simulink model "DisplayModel_Step3_start_harness"  (R2013b)
settings: Solver=FixedStepDiscrete  StartTime=0.0  StopTime=10.0  FixedStep=0.2  RelTol=1e-3
undefined symbols (not defined in the file): sigbuilder_block
libraries: simulink x1
settings Model: SldvGeneratedHarnessModel=TestUnitModel=DisplayModel_Step3_start|  CovMetricSettings=dcmoe  CovHTMLOptions=-aTS=1 -bRG=1 -bTC=0 -hTR=0 -nFC=0 -scm=1 -bcm=1  CovModelRefEnable=on  CovExternalEMLEnable=on  Creator=siddhars  LastModifiedBy=hualongy
settings DataIOCC: SaveFormat=StructureWithTime
settings OptimizationCC: ExpressionDepthLimit=2147483647  OptimizeModelRefInitCode=on  LifeSpan=1
settings DebuggingCC: InheritedTsInSrcMsg=none  StateNameClashWarn=warning
settings RTWCC: SystemTargetFile=ert.tlc  TemplateMakefile=ert_default_tmf  Description=Embedded Coder  ProcessScript=ert_make_rtw_hook  PortableWordSizes=on
settings CodeAppCC: IgnoreCustomStorageClasses=off  CustomSymbolStrType=$N$R$M  InternalIdentifier=Classic
settings ERTTargetCC: CodeReplacementLibrary=ANSI_C  GenerateSampleERTMain=on  ERTCustomFileTemplate=example_file_process.tlc
settings ConfigComp: Description=Design Verifier Custom Configuration Component  DVModelCoverageObjectives=MCDC  DVMaxTestCaseSteps=500  DVTestSuiteOptimization=CombinedObjectives (Nonlinear Extended)  DVSaveHarnessModel=on  DVModelReferenceHarness=on

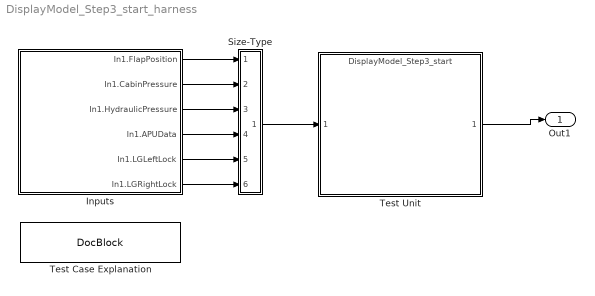
== system DisplayModel_Step3_start_harness ==
  Inputs : Subsystem  Tag=STV Subsys  LoadFcn=sigbuilder_block('load',[49.5 50.25 519.75 399.75 ]);  StartFcn=sigbuilder_block('start');  StopFcn=sigbuilder_block('stop');  ClipboardFcn=sigbuilder_block('clipboard');  mask(Sigbuilder block){}
      mask init:
      | if ~strcmp(get_param(bdroot(gcb),'SimulationStatus'),'stopped'),tuvar = sigbuilder_block('maskInit'); end
      settings: CopyFcn=sigbuilder_block('copy');  DeleteFcn=sigbuilder_block('delete');  ModelCloseFcn=sigbuilder_block('modelClose');  PreSaveFcn=sigbuilder_block('preSave');  PauseFcn=sigbuilder_block('pause');  ContinueFcn=sigbuilder_block('continue');  NameChangeFcn=sigbuilder_block('namechange');  OpenFcn=sigbuilder_block('open');  CloseFcn=sigbuilder_block('close');
      mask Display: plot(0, 0, 100, 100,[2, 2, 32, 32, 2], [68, 8, 8, 68, 68],[32, 2], [38, 38], [32, 19, 2],[53, 60, 44], [32, 17, 17, 2],[16, 16, 31, 31]);txt = getActiveGroup(gcbh);text(2, 100, txt,'verticalAlignment', 'top');
  Size-Type : Subsystem
  Test Case Explanation : simulink/Model-Wide Utilities/DocBlock  DocumentType=Text
  Test Unit : ModelReference  ModelNameDialog=DisplayModel_Step3_start  SimulationMode=Normal  ModelReferenceVersion=1.64  CopyOfModelName=DisplayModel_Step3_start  DefaultDataLogging=on
  Out1 : Outport
  wires:
  Inputs/1(In1.FlapPosition) -> Size-Type/1(In1)
  Inputs/2(In1.CabinPressure) -> Size-Type/2(In2)
  Inputs/3(In1.HydraulicPressure) -> Size-Type/3(In3)
  Inputs/4(In1.APUData) -> Size-Type/4(In4)
  Inputs/5(In1.LGLeftLock) -> Size-Type/5(In5)
  Inputs/6(In1.LGRightLock) -> Size-Type/6(In6)
  Size-Type/1(Out1) -> Test Unit/1
  Test Unit/1 -> Out1/1

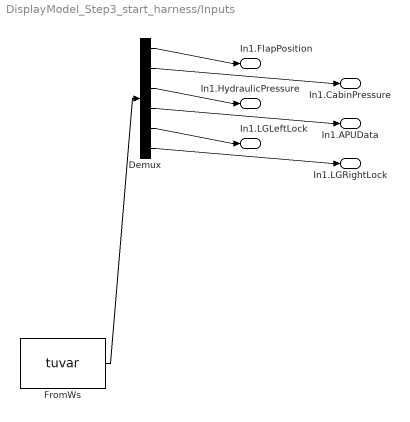
== system DisplayModel_Step3_start_harness/Inputs ==
  Demux : Demux  Tag=STV Demux  Outputs=6
  FromWs : FromWorkspace  Tag=STV FromWs  VariableName=tuvar  SampleTime=0
      SigBuilderData=|
      | dataSet.timeRange = [0 0.2]
      | dataSet.name = 'Test Case 1'
      | sbobj.Name = 'Signal Builder'
      | sbobj.Groups.Name = 'Test Case 1'
      | sbobj.Groups.Signals(1).Name = 'In1.FlapPosition'
      | sbobj.Groups.Signals(1).XData = [0 0.2]
      | sbobj.Groups.Signals(1).YData = [0 0]
      | sbobj.Groups.Signals(2).Name = 'In1.CabinPressure'
      | sbobj.Groups.Signals(2).XData = [0 0.2]
      | sbobj.Groups.Signals(2).YData = [0 0]
      | sbobj.Groups.Signals(3).Name = 'In1.HydraulicPressure'
      | sbobj.Groups.Signals(3).XData = [0 0.2]
      | sbobj.Groups.Signals(3).YData = [0 0]
      | sbobj.Groups.Signals(4).Name = 'In1.APUData'
      | sbobj.Groups.Signals(4).XData = [0 0.2]
      | sbobj.Groups.Signals(4).YData = [0 0]
      | sbobj.Groups.Signals(5).Name = 'In1.LGLeftLock'
      | sbobj.Groups.Signals(5).XData = [0 0.2]
      | sbobj.Groups.Signals(5).YData = [0 0]
      | sbobj.Groups.Signals(6).Name = 'In1.LGRightLock'
      | sbobj.Groups.Signals(6).XData = [0 0.2]
      | sbobj.Groups.Signals(6).YData = [0 0]
      | sbobj.Groups.TimeRange = [0 0.2]
  In1.FlapPosition : Outport  Tag=STV Outport
  In1.CabinPressure : Outport  Tag=STV Outport  Port=2
  In1.HydraulicPressure : Outport  Tag=STV Outport  Port=3
  In1.APUData : Outport  Tag=STV Outport  Port=4
  In1.LGLeftLock : Outport  Tag=STV Outport  Port=5
  In1.LGRightLock : Outport  Tag=STV Outport  Port=6
  wires:
  FromWs/1 -> Demux/1
  Demux/1 -> In1.FlapPosition/1
  Demux/2 -> In1.CabinPressure/1
  Demux/3 -> In1.HydraulicPressure/1
  Demux/4 -> In1.APUData/1
  Demux/5 -> In1.LGLeftLock/1
  Demux/6 -> In1.LGRightLock/1

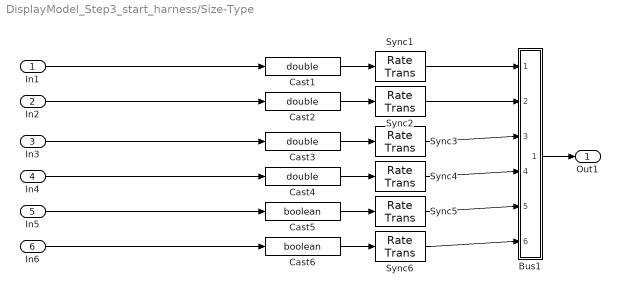
== system DisplayModel_Step3_start_harness/Size-Type ==
  In1 : Inport
  In2 : Inport  Port=2
  In3 : Inport  Port=3
  In4 : Inport  Port=4
  In5 : Inport  Port=5
  In6 : Inport  Port=6
  Bus1 : Subsystem
  Cast{1..4} (4 alike) : DataTypeConversion  OutDataTypeStr=double  SaturateOnIntegerOverflow=on  RndMeth=Zero
  Cast5 : DataTypeConversion  OutDataTypeStr=boolean  SaturateOnIntegerOverflow=on  RndMeth=Zero
  Cast6 : DataTypeConversion  OutDataTypeStr=boolean  SaturateOnIntegerOverflow=on  RndMeth=Zero
  Sync{1..6} (6 alike) : RateTransition  OutPortSampleTime=[0.20000000000000001,0]
  Out1 : Outport
  wires:
  In1/1 -> Cast1/1
  Cast1/1 -> Sync1/1
  In2/1 -> Cast2/1
  Cast2/1 -> Sync2/1
  In3/1 -> Cast3/1
  Cast3/1 -> Sync3/1
  In4/1 -> Cast4/1
  Cast4/1 -> Sync4/1
  In5/1 -> Cast5/1
  Cast5/1 -> Sync5/1
  In6/1 -> Cast6/1
  Cast6/1 -> Sync6/1
  Sync1/1 -> Bus1/1(In1(1).FlapPosition)
  Sync2/1 -> Bus1/2(In1(1).CabinPressure)
  Sync3/1 -> Bus1/3(In1(1).HydraulicPressure)
  Sync4/1 -> Bus1/4(In1(1).APUData)
  Sync5/1 -> Bus1/5(In1(1).LGLeftLock)
  Sync6/1 -> Bus1/6(In1(1).LGRightLock)
  Bus1/1(Out) -> Out1/1

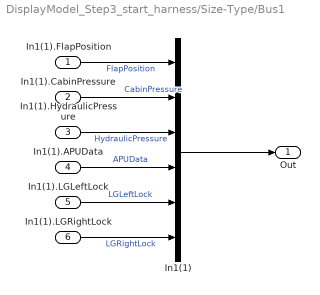
== system DisplayModel_Step3_start_harness/Size-Type/Bus1 ==
  In1(1).FlapPosition : Inport
  In1(1).CabinPressure : Inport  Port=2
  In1(1).HydraulicPressure : Inport  Port=3
  In1(1).APUData : Inport  Port=4
  In1(1).LGLeftLock : Inport  Port=5
  In1(1).LGRightLock : Inport  Port=6
  In1(1) : BusCreator  Inputs=6  OutDataTypeStr=Bus: MiscData
  Out : Outport
  wires:
  In1(1).FlapPosition/1 -> In1(1)/1  "FlapPosition"
  In1(1).CabinPressure/1 -> In1(1)/2  "CabinPressure"
  In1(1).HydraulicPressure/1 -> In1(1)/3  "HydraulicPressure"
  In1(1).APUData/1 -> In1(1)/4  "APUData"
  In1(1).LGLeftLock/1 -> In1(1)/5  "LGLeftLock"
  In1(1).LGRightLock/1 -> In1(1)/6  "LGRightLock"
  In1(1)/1 -> Out/1
